simulink model "Exercise1"  (R2025b)
settings: Solver=FixedStepAuto  StartTime=0.0  StopTime=300  FixedStep=Ts  RelTol=1e-3
values from neighbouring files (symbols this model uses):
  a = 0.923    [VehicleParameters.m]
  b = 1.376    [VehicleParameters.m]
  CMy = 0.1    [VehicleParameters.m]
  Cx = Cx0    [Exercise_Workbook.m]    (also in VehicleParameters.m = 0.33)
  Cz = 0.2    [VehicleParameters.m]
  eta_t = 0.93    [VehicleParameters.m]
  f0 = 0.011    [VehicleParameters.m]
  g = 9.81    [VehicleParameters.m]
  gear_vec = i_g    [Exercise_Workbook.m]
  ha = 0    [Exercise_Workbook.m]
  hb = 0.5    [Exercise_Workbook.m]
  hc = 0    [Exercise_Workbook.m]
  hG = 0.6    [VehicleParameters.m]
  i_f = 3.438    [VehicleParameters.m]
  i_g = [3.909 , 2.157 , 1.48 , 1.121 , 0.897]    [VehicleParameters.m]
  Je = 0.088    [VehicleParameters.m]
  Jt = 0.05    [VehicleParameters.m]
  Jw = 0.59    [VehicleParameters.m]
  K = 2.6e-8    (= 2.6e-08)    [VehicleParameters.m]
  l = a+b    (= 2.299)    [VehicleParameters.m]
  m = m0    [Exercise_Workbook.m]    (also in VehicleParameters.m = 1020)
  mu_vec = mu_wet    [Exercise_Workbook.m]
  n_shiftdown = 140    [Exercise_Workbook.m]
  n_shiftup = 450    [Exercise_Workbook.m]
  n_vec = n_compact    [Exercise_Workbook.m]
  omega0 = V0/Re    [Exercise_Workbook.m]
  Rc = Re    (= 0.279)    [VehicleParameters.m]
  ro = 1.2    [VehicleParameters.m]
  S = 2.04    [VehicleParameters.m]
  sigma_vec = sigma    [Exercise_Workbook.m]
  startingGear = 5    [Exercise_Workbook.m]
  t_pedalAct = 0.2    [Exercise_Workbook.m]
  t_shifting = 0.6    [Exercise_Workbook.m]
  T_vec = T_compact    [Exercise_Workbook.m]
  tau_f = 1./i_f    (= 0.290866783013)    [VehicleParameters.m]
  Tbf_max = TbTot/(1 + 1/Kb)    (= 2099.0990991)    [Exercise_Workbook.m]
  Tbr_max = Tbf_max/Kb    (= 900.900900901)    [Exercise_Workbook.m]
  Tc_max = 1.2*Te_max    (= 126)    [VehicleParameters.m]
  Traction = 2    [Exercise_Workbook.m]    (also in VehicleParameters.m = 1)
  Ts = 1e-3    (= 0.001)    [Exercise_Workbook.m]
  V0 = 80/3.6    (= 22.2222222222)    [Exercise_Workbook.m]
libraries: simulink x2
settings Model: Creator=Alberto  LastModifiedBy=denni
settings OptimizationCC: ReuseModelBlockBuffer=off
settings RTWCC: GPUComputeCapability=3.5

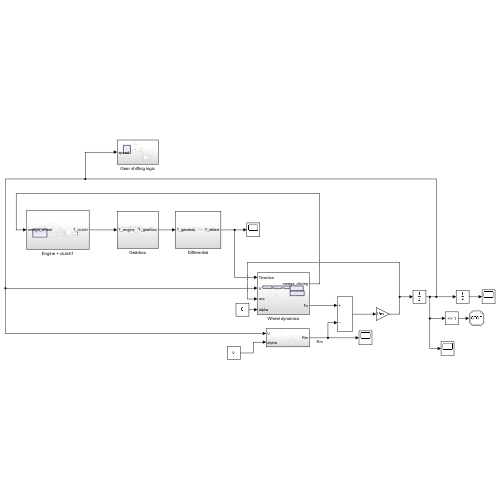
[thumbnail: Simulink's stored preview of the top-level diagram]
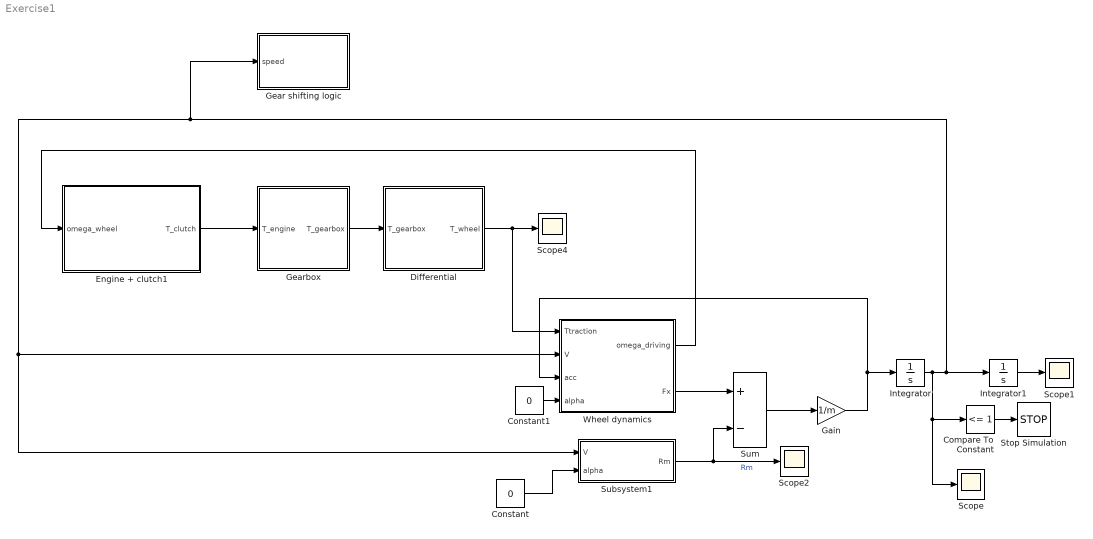
== system Exercise1 ==
  Compare To Constant : simulink/Logic and Bit Operations/Compare To Constant  relop=<=  const=1  OutDataTypeStr=boolean
  Constant : Constant  Value=0
  Constant1 : Constant  Value=0
  Differential : Subsystem
  Engine + clutch1 : Subsystem
  Gain : Gain  Gain=1/m
  Gear shifting logic : Subsystem
  Gearbox : Subsystem
  Integrator : Integrator  InitialCondition=V0
  Integrator1 : Integrator
  Scope{,1..2,4} (4 alike) : Scope
      Scope settings: ActiveDisplayYMinimum=-3.29722  ActiveDisplayYMaximum=4.84775  DataLoggingVariableName=Speed
      Scope1 settings: ActiveDisplayYMinimum=-21.94682  ActiveDisplayYMaximum=197.52142  DataLoggingVariableName=Distance
      Scope2 settings: ActiveDisplayYMinimum=-3.670379518302145E+57  ActiveDisplayYMaximum=3.3033415664719314E+58  DataLoggingVariableName=ScopeData3
      Scope4 settings: ActiveDisplayYMinimum=-433.41267  ActiveDisplayYMaximum=536.48619  DataLoggingVariableName=ScopeData9
  Stop Simulation : Stop
  Subsystem1 : Subsystem
  Sum : Sum  Inputs=+-
  Wheel dynamics : Subsystem
  wires:
  Integrator/1 -> Compare To Constant/1, Scope/1, Gear shifting logic/1(speed), Wheel dynamics/2(V), Subsystem1/1(V), Integrator1/1
  Wheel dynamics/2(Fx) -> Sum/1
  Subsystem1/1(Rm) -> Scope2/1, Sum/2  "Rm"
  Constant/1 -> Subsystem1/2(alpha)
  Sum/1 -> Gain/1
  Gain/1 -> Wheel dynamics/3(acc), Integrator/1
  Integrator1/1 -> Scope1/1
  Compare To Constant/1 -> Stop Simulation/1
  Constant1/1 -> Wheel dynamics/4(alpha)
  Gearbox/1(T_gearbox) -> Differential/1(T_gearbox)
  Differential/1(T_wheel) -> Wheel dynamics/1(Ttraction), Scope4/1
  Engine + clutch1/1(T_clutch) -> Gearbox/1(T_engine)
  Wheel dynamics/1(omega_driving) -> Engine + clutch1/1(omega_wheel)

== system Exercise1/Differential ==
  T_gearbox : Inport
  Gain3 : Gain  Gain=0.5*i_f
  T_wheel : Outport
  wires:
  T_gearbox/1 -> Gain3/1
  Gain3/1 -> T_wheel/1

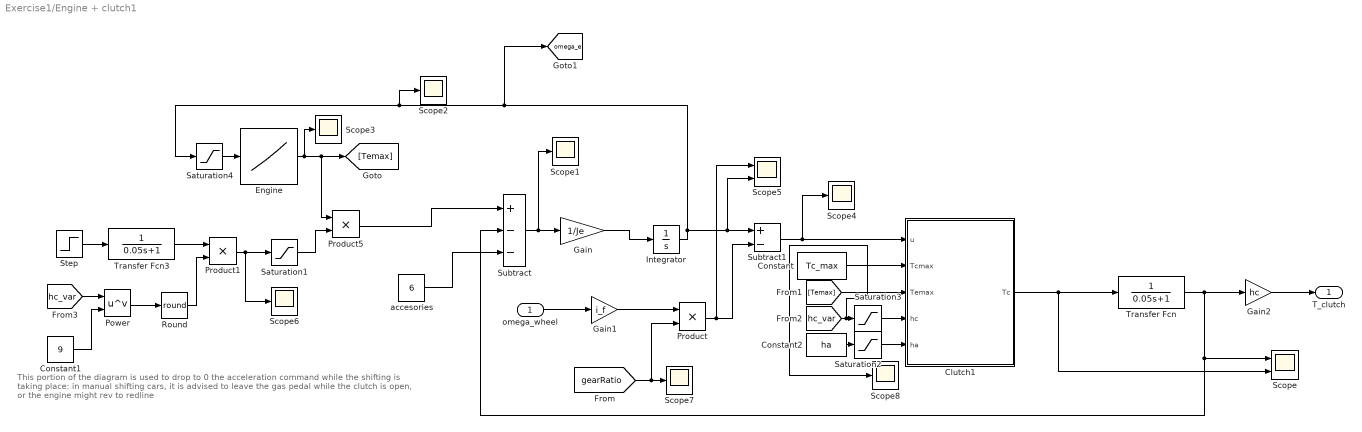
== system Exercise1/Engine + clutch1 ==
  note: This portion of the diagram is used to drop to 0 the acceleration command while the shifting is taking place: in manual shifting cars, it is advised to leave the gas pedal while the clutch is open, or the engine might rev to redline
  omega_wheel : Inport
  Clutch1 : MATLAB Function  TreatAsAtomicUnit=on
  Constant : Constant  Value=Tc_max
  Constant1 : Constant  Value=9
  Constant2 : Constant  Value=ha
  Engine : Lookup_n-D  NumberOfTableDimensions=1  BreakpointsForDimension1=n_vec  Table=T_vec  InternalRulePriority=Speed  RndMeth=Simplest
  Gain : Gain  Gain=1/Je
  Gain1 : Gain  Gain=i_f
  Gain2 : Gain  Gain=hc
  Integrator : Integrator  InitialCondition=omega0*i_g(5)*i_f
  Power : Math  Operator=pow
  Product : Product
  Product1 : Product
  Product5 : Product
  Round : Rounding  Operator=round
  Saturation1 : Saturate  UpperLimit=1  LowerLimit=0
  Saturation2 : Saturate  UpperLimit=1  LowerLimit=0
  Saturation3 : Saturate  UpperLimit=1  LowerLimit=0
  Saturation4 : Saturate  UpperLimit=max(n_vec)  LowerLimit=min(n_vec)
  Scope : Scope  NumInputPorts=2
      settings: ActiveDisplayYMinimum=-157.5  ActiveDisplayYMaximum=157.5  DataLoggingVariableName=ScopeData11
  Scope{1..4,6..8} (7 alike) : Scope
      Scope1 settings: ActiveDisplayYMinimum=-1.4800422611786087E+307  ActiveDisplayYMaximum=1.6444914013095649E+306  DataLoggingVariableName=ScopeData5
      Scope2 settings: ActiveDisplayYMinimum=-234.98976  ActiveDisplayYMaximum=2163.66995  DataLoggingVariableName=ScopeData6
      Scope3 settings: ActiveDisplayYMinimum=42.3058  ActiveDisplayYMaximum=110.8549  DataLoggingVariableName=ScopeData7
      Scope4 settings: ActiveDisplayYMinimum=-233.77506  ActiveDisplayYMaximum=296.88623  DataLoggingVariableName=ScopeData9
      Scope6 settings: ActiveDisplayYMinimum=-1  ActiveDisplayYMaximum=1
      Scope7 settings: ActiveDisplayYMinimum=3.85912  ActiveDisplayYMaximum=3.95022  DataLoggingVariableName=ScopeData2
      Scope8 settings: ActiveDisplayYMinimum=-0.11944  ActiveDisplayYMaximum=1.12438  DataLoggingVariableName=ScopeData2
  Scope5 : Scope  NumInputPorts=2
      settings: ActiveDisplayYMinimum=-55.03177  ActiveDisplayYMaximum=558.78238  DataLoggingVariableName=ScopeData10
  Step : Step  Time=0  After=ha  SampleTime=0
  Subtract : Sum  Inputs=+--
  Subtract1 : Sum  Inputs=+-
  Transfer Fcn : TransferFcn  Denominator=[0.05 1]
  Transfer Fcn3 : TransferFcn  Denominator=[0.05 1]
  accesories : Constant  Value=6
  T_clutch : Outport
  tag scope: omega_e=global
  wires:
  Engine/1 -> Scope3/1, [Temax], Product5/1
  Product5/1 -> Subtract/1
  Saturation1/1 -> Product5/2
  Subtract/1 -> Scope1/1, Gain/1
  Gain/1 -> Integrator/1
  omega_wheel/1 -> Gain1/1
  Gain1/1 -> Product/1
  [gearRatio] -> Product/2, Scope7/1
  Product/1 -> Scope5/1, Subtract1/2
  Subtract1/1 -> Clutch1/1(u), Scope4/1
  Constant/1 -> Clutch1/2(Tcmax)
  [Temax] -> Clutch1/3(Temax)
  Saturation3/1 -> Clutch1/4(hc)
  [hc_var] -> Scope8/1, Saturation3/1
  Constant2/1 -> Saturation2/1
  Saturation2/1 -> Clutch1/5(ha)
  Integrator/1 -> [omega_e], Saturation4/1, Scope2/1, Scope5/2, Subtract1/1
  Transfer Fcn3/1 -> Product1/1
  Product1/1 -> Scope6/1, Saturation1/1
  Round/1 -> Product1/2
  [hc_var] -> Power/1
  Power/1 -> Round/1
  Constant1/1 -> Power/2
  Clutch1/1(Tc) -> Scope/2, Transfer Fcn/1
  Step/1 -> Transfer Fcn3/1
  Saturation4/1 -> Engine/1
  accesories/1 -> Subtract/3
  Gain2/1 -> T_clutch/1
  Transfer Fcn/1 -> Subtract/2, Scope/1, Gain2/1

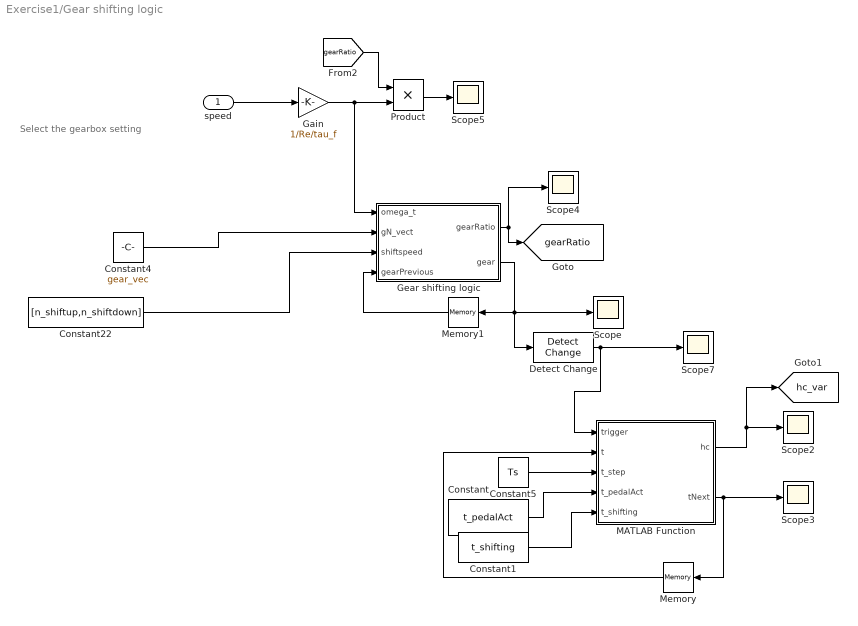
== system Exercise1/Gear shifting logic ==
  note: Select the gearbox setting
  speed : Inport
  Constant : Constant  Value=t_pedalAct
  Constant1 : Constant  Value=t_shifting
  Constant22 : Constant  Value=[n_shiftup,n_shiftdown]
  Constant4 : Constant  Value=gear_vec  SampleTime=Ts
  Constant5 : Constant  Value=Ts
  Detect Change : simulink/Logic and Bit Operations/Detect Change  vinit=0  OutDataTypeStr=boolean
  Gain : Gain  Gain=1/Re/tau_f
  Gear shifting logic : MATLAB Function  TreatAsAtomicUnit=on
  MATLAB Function : MATLAB Function  TreatAsAtomicUnit=on
  Memory : Memory
  Memory1 : Memory  InitialCondition=startingGear
  Product : Product
  Scope{,2..5,7} (6 alike) : Scope
      Scope settings: ActiveDisplayYMinimum=0.5  ActiveDisplayYMaximum=5.5
      Scope2 settings: ActiveDisplayYMinimum=-0.11944  ActiveDisplayYMaximum=1.12438  DataLoggingVariableName=ScopeData2
      Scope3 settings: ActiveDisplayYMinimum=-0.6325  ActiveDisplayYMaximum=5.6925  DataLoggingVariableName=ScopeData3
      Scope4 settings: ActiveDisplayYMinimum=0.7725  ActiveDisplayYMaximum=4.2575  DataLoggingVariableName=ScopeData8
      Scope5 settings: ActiveDisplayYMinimum=-25.93069  ActiveDisplayYMaximum=467.45559
      Scope7 settings: ActiveDisplayYMinimum=-0.125  ActiveDisplayYMaximum=1.125  DataLoggingVariableName=ScopeData2
  tag scope: gearRatio=global, hc_var=global
  wires:
  Gear shifting logic/1(gearRatio) -> [gearRatio], Scope4/1
  Constant22/1 -> Gear shifting logic/3(shiftspeed)
  Gear shifting logic/2(gear) -> Scope/1, Memory1/1, Detect Change/1
  Detect Change/1 -> MATLAB Function/1(trigger), Scope7/1
  MATLAB Function/2(tNext) -> Scope3/1, Memory/1
  Memory/1 -> MATLAB Function/2(t)
  MATLAB Function/1(hc) -> [hc_var], Scope2/1
  Memory1/1 -> Gear shifting logic/4(gearPrevious)
  Constant/1 -> MATLAB Function/4(t_pedalAct)
  Constant1/1 -> MATLAB Function/5(t_shifting)
  Constant5/1 -> MATLAB Function/3(t_step)
  speed/1 -> Gain/1
  Gain/1 -> Product/2, Gear shifting logic/1(omega_t)
  Constant4/1 -> Gear shifting logic/2(gN_vect)
  [gearRatio] -> Product/1
  Product/1 -> Scope5/1

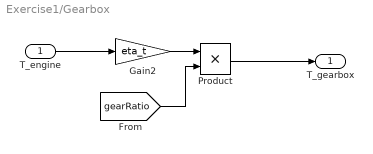
== system Exercise1/Gearbox ==
  T_engine : Inport
  Gain2 : Gain  Gain=eta_t
  Product : Product
  T_gearbox : Outport
  wires:
  Gain2/1 -> Product/1
  T_engine/1 -> Gain2/1
  Product/1 -> T_gearbox/1
  [gearRatio] -> Product/2

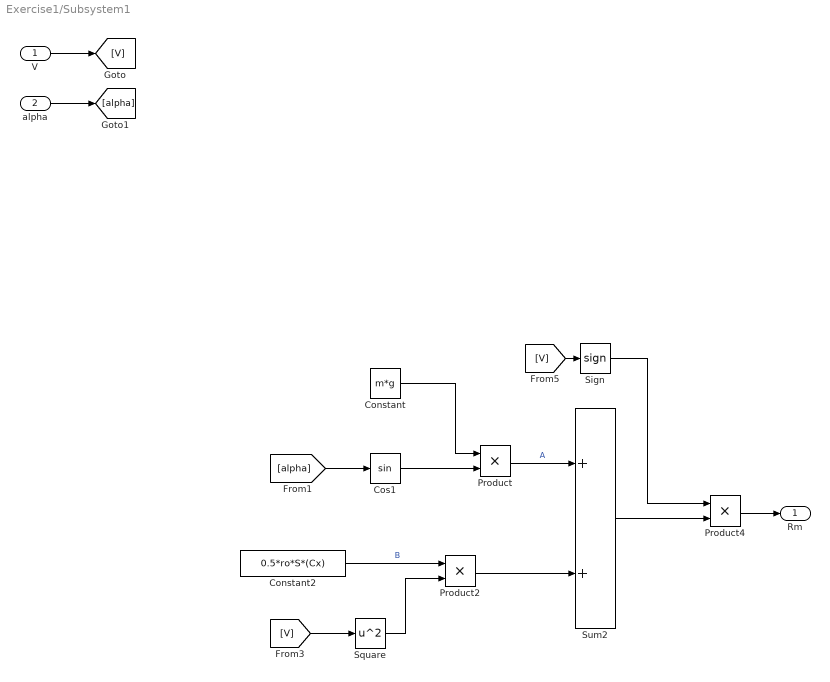
== system Exercise1/Subsystem1 ==
  V : Inport
  alpha : Inport  Port=2
  Constant : Constant  Value=m*g
  Constant2 : Constant  Value=0.5*ro*S*(Cx)
  Cos1 : Trigonometry
  Product : Product
  Product2 : Product
  Product4 : Product
  Sign : Signum
  Square : Math  Operator=square
  Sum2 : Sum
  Rm : Outport
  wires:
  V/1 -> [V]
  alpha/1 -> [alpha]
  [alpha] -> Cos1/1
  Cos1/1 -> Product/2
  Constant/1 -> Product/1
  Product/1 -> Sum2/1  "A"
  Constant2/1 -> Product2/1  "B"
  [V] -> Square/1
  Square/1 -> Product2/2
  Product2/1 -> Sum2/2
  Product4/1 -> Rm/1
  Sum2/1 -> Product4/2
  [V] -> Sign/1
  Sign/1 -> Product4/1

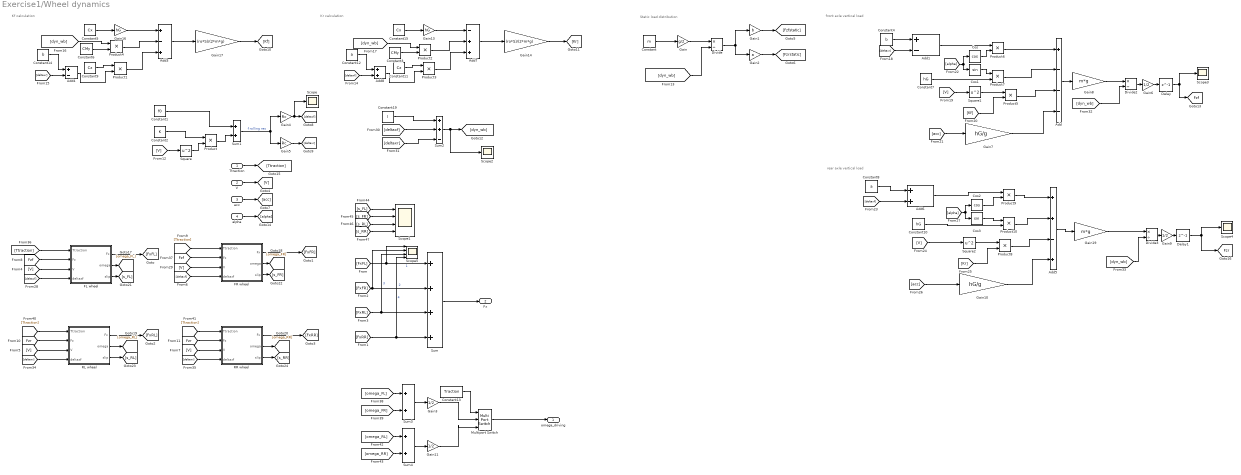
== system Exercise1/Wheel dynamics ==
  note: Static load distribution
  note: Kr calculation
  note: Kf calculation
  note: front axle vertical load
  note: rear axle vertical load
  Ttraction : Inport
  V : Inport  Port=2
  acc : Inport  Port=3
  alpha : Inport  Port=4
  Add : Sum  Inputs=+---
  Add1 : Sum  Inputs=+-
  Add3 : Sum  Inputs=+-+
  Add4 : Sum  Inputs=+-
  Add5 : Sum  Inputs=++-+
  Add6 : Sum
  Add7 : Sum  Inputs=-++
  Add8 : Sum
  Constant : Constant  Value=m
  Constant1 : Constant  Value=f0
  Constant10 : Constant  Value=hG
  Constant11 : Constant  Value=Cz
  Constant12 : Constant  Value=a
  Constant13 : Constant  Value=Traction
  Constant14 : Constant  Value=b
  Constant15 : Constant  Value=Cx
  Constant19 : Constant  Value=l
  Constant2 : Constant  Value=K
  Constant3 : Constant  Value=CMy
  Constant4 : Constant  Value=b
  Constant5 : Constant  Value=Cx
  Constant6 : Constant  Value=CMy
  Constant7 : Constant  Value=hG
  Constant8 : Constant  Value=a
  Constant9 : Constant  Value=Cz
  Cos : Trigonometry  Operator=cos
  Cos1 : Trigonometry
  Cos2 : Trigonometry  Operator=cos
  Cos3 : Trigonometry
  Delay : Delay  DelayLength=1  InitialCondition=m*g*b/l/2
  Delay1 : Delay  DelayLength=1  InitialCondition=m*g*a/l/2
  Divide : Product  Inputs=*/
  Divide2 : Product  Inputs=*/
  Divide3 : Product  Inputs=*/
  FL wheel : Subsystem
  FR wheel : Subsystem
  Gain : Gain  Gain=g/2
  Gain1 : Gain  Gain=b
  Gain10 : Gain  Gain=hG/g
  Gain{3,6,9,11} (4 alike) : Gain  Gain=1/2
  Gain13 : Gain  Gain=hG
  Gain14 : Gain  Gain=(ro*S)/(2*m*g)
  Gain16 : Gain  Gain=hG
  Gain17 : Gain  Gain=(ro*S)/(2*m*g)
  Gain19 : Gain  Gain=m*g
  Gain2 : Gain  Gain=a
  Gain4 : Gain  Gain=Rc
  Gain5 : Gain  Gain=Rc
  Gain7 : Gain  Gain=hG/g
  Gain8 : Gain  Gain=m*g
  Multiport Switch : MultiPortSwitch  Inputs=2  SaturateOnIntegerOverflow=off  InputSameDT=off
  Product{,1..10} (11 alike) : Product
  RL wheel : Subsystem
  RR wheel : Subsystem
  Scope{,2..4} (4 alike) : Scope
      Scope settings: ActiveDisplayYMinimum=0.003067  ActiveDisplayYMaximum=0.003086  DataLoggingVariableName=ScopeData2
      Scope2 settings: ActiveDisplayYMinimum=1.299  ActiveDisplayYMaximum=3.299  DataLoggingVariableName=ScopeData4
      Scope3 settings: ActiveDisplayYMinimum=2850.0417  ActiveDisplayYMaximum=3925.07758
      Scope4 settings: ActiveDisplayYMinimum=1017.63681  ActiveDisplayYMaximum=2054.66126  DataLoggingVariableName=ScopeData2
  Scope1 : Scope  NumInputPorts=4
      settings: ActiveDisplayYMinimum=-0.57113  ActiveDisplayYMaximum=0.11334  DataLoggingVariableName=slip
  Scope5 : Scope  NumInputPorts=4
      settings: ActiveDisplayYMinimum=-3828.18796  ActiveDisplayYMaximum=425.35422  DataLoggingVariableName=ScopeData3
  Square : Math  Operator=square
  Square1 : Math  Operator=square
  Square2 : Math  Operator=square
  Sum : Sum  Inputs=++++
  Sum1 : Sum
  Sum2 : Sum  Inputs=++-
  Sum3 : Sum
  Sum4 : Sum
  omega_driving : Outport
  Fx : Outport  Port=2
  tag scope: Fzf=global, Fzr=global
  wires:
  FL wheel/1(Fx) -> [FxFL]
  [V] -> RR wheel/3(V)
  [FxRL] -> Scope5/3, Sum/3  "3"
  V/1 -> [V]
  Sum/1 -> Fx/1
  RR wheel/1(Fx) -> [FxRR]
  [FxRR] -> Scope5/4, Sum/4  "4"
  [FxFL] -> Scope5/1, Sum/1  "1"
  FR wheel/1(Fx) -> [FxFR]
  [V] -> FL wheel/3(V)
  [V] -> RL wheel/3(V)
  RL wheel/1(Fx) -> [FxRL]
  [Fzf] -> FL wheel/2(Fz)
  Constant/1 -> Gain/1
  Gain1/1 -> [Fzfstatic]
  Gain2/1 -> [Fzrstatic]
  [Fzr] -> RL wheel/2(Fz)
  [Fzr] -> RR wheel/2(Fz)
  acc/1 -> [acc]
  [V] -> Square/1
  Constant2/1 -> Product/1
  Square/1 -> Product/2
  Constant1/1 -> Sum1/1
  Product/1 -> Sum1/2
  Sum1/1 -> Gain5/1, Gain4/1  "f rolling res"
  Gain4/1 -> Scope/1, [deltaxf]
  Gain5/1 -> [deltaxr]
  Constant19/1 -> Sum2/1
  [deltaxr] -> Sum2/3
  Sum2/1 -> Scope2/1, [dyn_wb]
  [deltaxf] -> Sum2/2
  Gain/1 -> Divide/1
  [dyn_wb] -> Divide/2
  Divide/1 -> Gain2/1, Gain1/1
  Add4/1 -> Product1/2
  Gain17/1 -> [Kf]
  Product1/1 -> Add3/3
  Product3/1 -> Add7/3
  Constant5/1 -> Gain16/1
  Add8/1 -> Product3/2
  Constant12/1 -> Add8/1
  Constant15/1 -> Gain13/1
  Product2/1 -> Add7/2
  Product4/1 -> Add3/2
  Add3/1 -> Gain17/1
  Constant9/1 -> Product1/1
  Constant11/1 -> Product3/1
  [deltaxr] -> Add4/2
  Add7/1 -> Gain14/1
  Gain14/1 -> [Kr]
  [deltaxf] -> Add8/2
  Gain13/1 -> Add7/1
  Gain16/1 -> Add3/1
  Constant14/1 -> Add4/1
  Constant6/1 -> Product4/2
  [dyn_wb] -> Product4/1
  Constant3/1 -> Product2/2
  [dyn_wb] -> Product2/1
  Product5/1 -> Add/3
  Gain7/1 -> Add/4
  Square1/1 -> Product5/1
  Constant4/1 -> Add1/1
  [Kf] -> Product5/2
  Product7/1 -> Add/2
  Add1/1 -> Product6/1
  Constant7/1 -> Product7/2
  [dyn_wb] -> Divide2/2
  [V] -> Square1/1
  [acc] -> Gain7/1
  Gain8/1 -> Divide2/1
  Product6/1 -> Add/1
  Add/1 -> Gain8/1
  [deltaxr] -> Add1/2
  Cos/1 -> Product6/2
  Cos1/1 -> Product7/1
  alpha/1 -> [alpha]
  [alpha] -> Cos/1, Cos1/1
  Divide2/1 -> Gain6/1
  [V] -> Square2/1
  [acc] -> Gain10/1
  Constant10/1 -> Product10/2
  Add5/1 -> Gain19/1
  Constant8/1 -> Add6/1
  Product9/1 -> Add5/1
  [dyn_wb] -> Divide3/2
  Add6/1 -> Product9/1
  Square2/1 -> Product8/1
  Product8/1 -> Add5/3
  [Kr] -> Product8/2
  Gain19/1 -> Divide3/1
  Gain10/1 -> Add5/4
  Product10/1 -> Add5/2
  [deltaxf] -> Add6/2
  [alpha] -> Cos2/1, Cos3/1
  Cos2/1 -> Product9/2
  Cos3/1 -> Product10/1
  Divide3/1 -> Gain9/1
  Gain6/1 -> Delay/1
  Delay/1 -> [Fzf], Scope3/1
  Gain9/1 -> Delay1/1
  [deltaxf] -> FL wheel/4(deltaxf)
  [deltaxr] -> RL wheel/4(deltaxf)
  [deltaxr] -> RR wheel/4(deltaxf)
  Delay1/1 -> [Fzr], Scope4/1
  Ttraction/1 -> [Ttraction]
  [Ttraction] -> FL wheel/1(Ttraction)
  [Ttraction] -> FR wheel/1(Ttraction)
  [V] -> FR wheel/3(V)
  [deltaxf] -> FR wheel/4(deltaxf)
  [Fzf] -> FR wheel/2(Fz)
  FL wheel/2(omega) -> [omega_FL]
  FR wheel/2(omega) -> [omega_FR]
  [omega_FL] -> Sum3/1
  [omega_FR] -> Sum3/2
  Sum3/1 -> Gain3/1
  [Ttraction] -> RL wheel/1(Ttraction)
  RL wheel/2(omega) -> [omega_RL]
  [Ttraction] -> RR wheel/1(Ttraction)
  RR wheel/2(omega) -> [omega_RR]
  Sum4/1 -> Gain11/1
  [omega_RR] -> Sum4/2
  [omega_RL] -> Sum4/1
  Gain3/1 -> Multiport Switch/2
  Gain11/1 -> Multiport Switch/3
  Constant13/1 -> Multiport Switch/1
  Multiport Switch/1 -> omega_driving/1
  FL wheel/3(slip) -> [s_FL]
  FR wheel/3(slip) -> [s_FR]
  RL wheel/3(slip) -> [s_RL]
  RR wheel/3(slip) -> [s_RR]
  [s_FL] -> Scope1/1
  [s_FR] -> Scope1/2
  [s_RL] -> Scope1/3
  [s_RR] -> Scope1/4
  [FxFR] -> Scope5/2, Sum/2  "2"

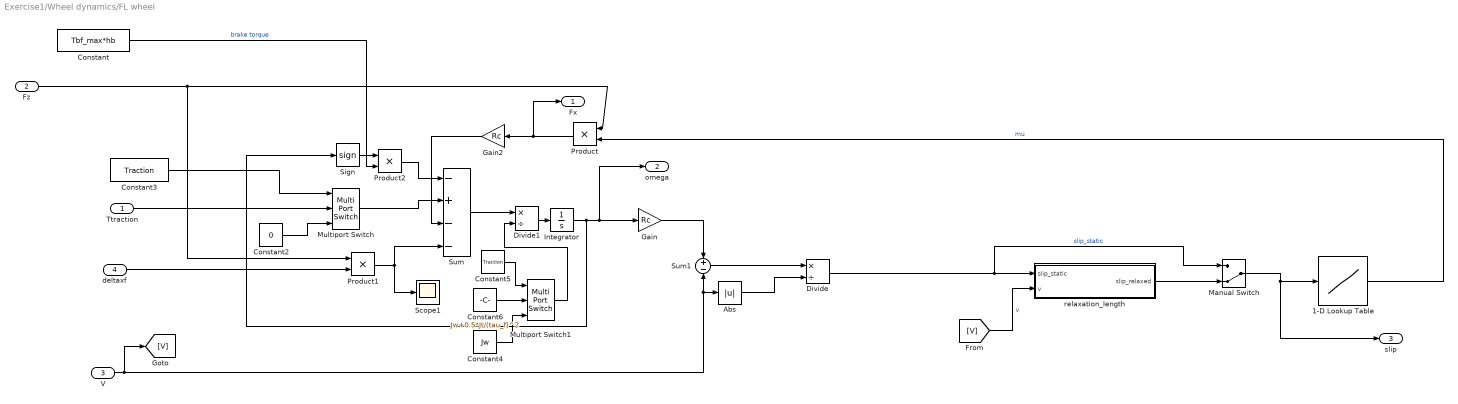
== system Exercise1/Wheel dynamics/FL wheel ==
  Ttraction : Inport
  Fz : Inport  Port=2
  V : Inport  Port=3
  deltaxf : Inport  Port=4
  1-D Lookup Table : Lookup_n-D  NumberOfTableDimensions=1  BreakpointsForDimension1=sigma_vec  Table=mu_vec  InternalRulePriority=Speed  RndMeth=Simplest
  Abs : Abs  SaturateOnIntegerOverflow=off
  Constant : Constant  Value=Tbf_max*hb
  Constant2 : Constant  Value=0
  Constant3 : Constant  Value=Traction
  Constant4 : Constant  Value=Jw
  Constant5 : Constant  Value=Traction
  Constant6 : Constant  Value=Jw+0.5*Jt/(tau_f)^2
  Divide : Product  Inputs=*/
  Divide1 : Product  Inputs=*/
  Gain : Gain  Gain=Rc
  Gain2 : Gain  Gain=Rc
  Integrator : Integrator  InitialCondition=omega0  LimitOutput=on  LowerSaturationLimit=0
  Manual Switch : ManualSwitch  CurrentSetting=0
  Multiport Switch : MultiPortSwitch  Inputs=2  SaturateOnIntegerOverflow=off  InputSameDT=off
  Multiport Switch1 : MultiPortSwitch  Inputs=2  SaturateOnIntegerOverflow=off  InputSameDT=off
  Product : Product
  Product1 : Product
  Product2 : Product
  Scope1 : Scope
      settings: ActiveDisplayYMinimum=4.6511  ActiveDisplayYMaximum=15.35009  DataLoggingVariableName=ScopeData8
  Sign : Signum
  Sum : Sum  Inputs=-+--
  Sum1 : Sum  Inputs=+-
  relaxation_length : Subsystem
  Fx : Outport
  omega : Outport  Port=2
  slip : Outport  Port=3
  wires:
  Gain/1 -> Sum1/1
  Gain2/1 -> Sum/3
  V/1 -> [V], Abs/1, Sum1/2
  Product/1 -> Fx/1, Gain2/1
  1-D Lookup Table/1 -> Product/2  "mu"
  Integrator/1 -> Sign/1, omega/1, Gain/1
  Sum1/1 -> Divide/1
  Divide/1 -> relaxation_length/1(slip_static), Manual Switch/1  "slip_static"
  Fz/1 -> Product/1, Product1/1
  Abs/1 -> Divide/2
  deltaxf/1 -> Product1/2
  Product1/1 -> Sum/4, Scope1/1
  Multiport Switch/1 -> Sum/2
  Constant2/1 -> Multiport Switch/3
  Ttraction/1 -> Multiport Switch/2
  Constant3/1 -> Multiport Switch/1
  Constant5/1 -> Multiport Switch1/1
  Multiport Switch1/1 -> Divide1/2
  Sum/1 -> Divide1/1
  Constant4/1 -> Multiport Switch1/3
  Constant6/1 -> Multiport Switch1/2
  Divide1/1 -> Integrator/1
  Sign/1 -> Product2/1
  Constant/1 -> Product2/2  "brake torque"
  Product2/1 -> Sum/1
  [V] -> relaxation_length/2(v)  "v"
  Manual Switch/1 -> slip/1, 1-D Lookup Table/1
  relaxation_length/1(slip_relaxed) -> Manual Switch/2

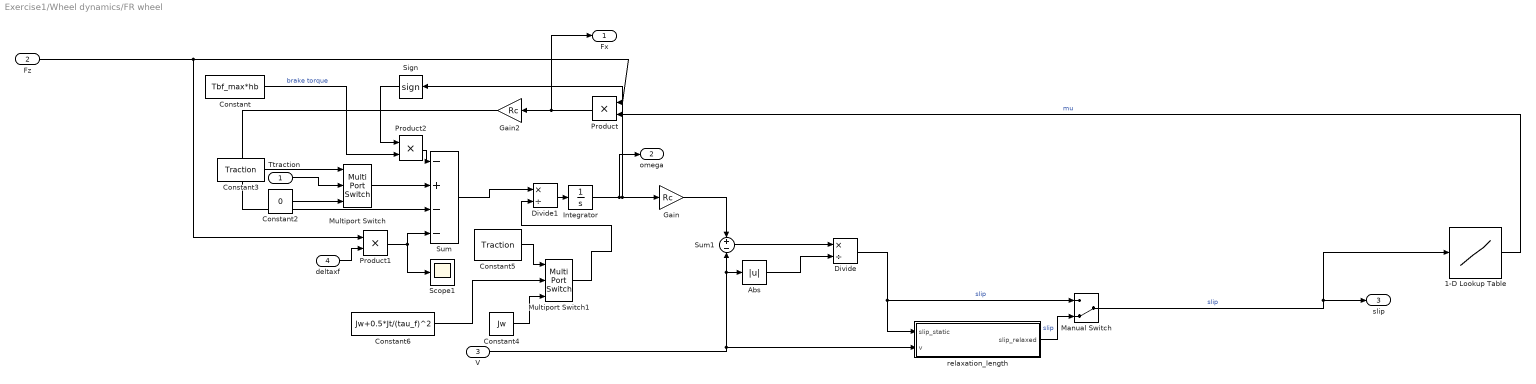
== system Exercise1/Wheel dynamics/FR wheel ==
  Ttraction : Inport
  Fz : Inport  Port=2
  V : Inport  Port=3
  deltaxf : Inport  Port=4
  1-D Lookup Table : Lookup_n-D  NumberOfTableDimensions=1  BreakpointsForDimension1=sigma_vec  Table=mu_vec  InternalRulePriority=Speed  RndMeth=Simplest
  Abs : Abs  SaturateOnIntegerOverflow=off
  Constant : Constant  Value=Tbf_max*hb
  Constant2 : Constant  Value=0
  Constant3 : Constant  Value=Traction
  Constant4 : Constant  Value=Jw
  Constant5 : Constant  Value=Traction
  Constant6 : Constant  Value=Jw+0.5*Jt/(tau_f)^2
  Divide : Product  Inputs=*/
  Divide1 : Product  Inputs=*/
  Gain : Gain  Gain=Rc
  Gain2 : Gain  Gain=Rc
  Integrator : Integrator  InitialCondition=omega0  LimitOutput=on  LowerSaturationLimit=0
  Manual Switch : ManualSwitch  CurrentSetting=0
  Multiport Switch : MultiPortSwitch  Inputs=2  SaturateOnIntegerOverflow=off  InputSameDT=off
  Multiport Switch1 : MultiPortSwitch  Inputs=2  SaturateOnIntegerOverflow=off  InputSameDT=off
  Product : Product
  Product1 : Product
  Product2 : Product
  Scope1 : Scope
      settings: ActiveDisplayYMinimum=4.6511  ActiveDisplayYMaximum=15.35009  DataLoggingVariableName=ScopeData8
  Sign : Signum
  Sum : Sum  Inputs=-+--
  Sum1 : Sum  Inputs=+-
  relaxation_length : Subsystem
  Fx : Outport
  omega : Outport  Port=2
  slip : Outport  Port=3
  wires:
  Product2/1 -> Sum/1
  Constant/1 -> Product2/2  "brake torque"
  Sign/1 -> Product2/1
  Divide1/1 -> Integrator/1
  Constant6/1 -> Multiport Switch1/2
  Constant4/1 -> Multiport Switch1/3
  Sum/1 -> Divide1/1
  Multiport Switch1/1 -> Divide1/2
  Constant5/1 -> Multiport Switch1/1
  Constant3/1 -> Multiport Switch/1
  Ttraction/1 -> Multiport Switch/2
  Constant2/1 -> Multiport Switch/3
  Multiport Switch/1 -> Sum/2
  Product1/1 -> Scope1/1, Sum/4
  deltaxf/1 -> Product1/2
  Abs/1 -> Divide/2
  Fz/1 -> Product1/1, Product/1
  Manual Switch/1 -> 1-D Lookup Table/1, slip/1  "slip"
  Sum1/1 -> Divide/1
  Integrator/1 -> Sign/1, Gain/1, omega/1
  1-D Lookup Table/1 -> Product/2  "mu"
  Product/1 -> Gain2/1, Fx/1
  V/1 -> relaxation_length/2(v), Sum1/2, Abs/1
  Gain2/1 -> Sum/3
  Gain/1 -> Sum1/1
  Divide/1 -> relaxation_length/1(slip_static), Manual Switch/1  "slip"
  relaxation_length/1(slip_relaxed) -> Manual Switch/2  "slip"

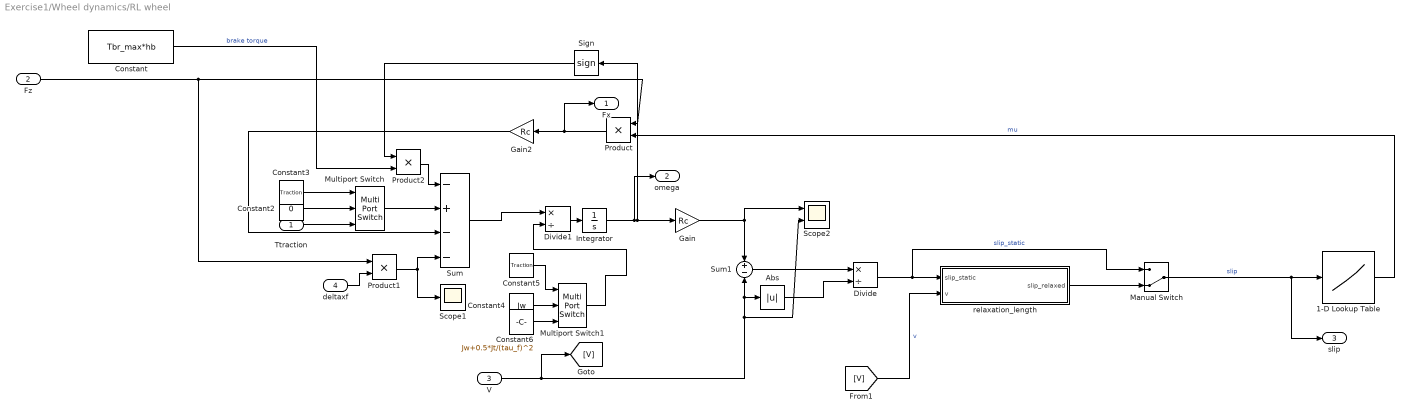
== system Exercise1/Wheel dynamics/RL wheel ==
  Ttraction : Inport
  Fz : Inport  Port=2
  V : Inport  Port=3
  deltaxf : Inport  Port=4
  1-D Lookup Table : Lookup_n-D  NumberOfTableDimensions=1  BreakpointsForDimension1=sigma_vec  Table=mu_vec  InternalRulePriority=Speed  RndMeth=Simplest
  Abs : Abs  SaturateOnIntegerOverflow=off
  Constant : Constant  Value=Tbr_max*hb
  Constant2 : Constant  Value=0
  Constant3 : Constant  Value=Traction
  Constant4 : Constant  Value=Jw
  Constant5 : Constant  Value=Traction
  Constant6 : Constant  Value=Jw+0.5*Jt/(tau_f)^2
  Divide : Product  Inputs=*/
  Divide1 : Product  Inputs=*/
  Gain : Gain  Gain=Rc
  Gain2 : Gain  Gain=Rc
  Integrator : Integrator  InitialCondition=omega0  LimitOutput=on  LowerSaturationLimit=0
  Manual Switch : ManualSwitch  CurrentSetting=0
  Multiport Switch : MultiPortSwitch  Inputs=2  SaturateOnIntegerOverflow=off  InputSameDT=off
  Multiport Switch1 : MultiPortSwitch  Inputs=2  SaturateOnIntegerOverflow=off  InputSameDT=off
  Product : Product
  Product1 : Product
  Product2 : Product
  Scope1 : Scope
      settings: ActiveDisplayYMinimum=1.38626  ActiveDisplayYMaximum=12.08532  DataLoggingVariableName=ScopeData8
  Scope2 : Scope  NumInputPorts=2
      settings: ActiveDisplayYMinimum=-5.63176  ActiveDisplayYMaximum=50.62575  DataLoggingVariableName=ScopeData6
  Sign : Signum
  Sum : Sum  Inputs=-+--
  Sum1 : Sum  Inputs=+-
  relaxation_length : Subsystem
  Fx : Outport
  omega : Outport  Port=2
  slip : Outport  Port=3
  wires:
  Gain/1 -> Sum1/1, Scope2/1
  Gain2/1 -> Sum/3
  V/1 -> [V], Sum1/2, Abs/1, Scope2/2
  Product/1 -> Fx/1, Gain2/1
  1-D Lookup Table/1 -> Product/2  "mu"
  Integrator/1 -> Sign/1, Gain/1, omega/1
  Sum1/1 -> Divide/1
  Manual Switch/1 -> slip/1, 1-D Lookup Table/1  "slip"
  Fz/1 -> Product/1, Product1/1
  deltaxf/1 -> Product1/2
  Product1/1 -> Sum/4, Scope1/1
  Multiport Switch/1 -> Sum/2
  Constant3/1 -> Multiport Switch/1
  Constant5/1 -> Multiport Switch1/1
  Multiport Switch1/1 -> Divide1/2
  Sum/1 -> Divide1/1
  Divide1/1 -> Integrator/1
  Constant6/1 -> Multiport Switch1/3
  Constant4/1 -> Multiport Switch1/2
  Constant2/1 -> Multiport Switch/2
  Ttraction/1 -> Multiport Switch/3
  Product2/1 -> Sum/1
  Sign/1 -> Product2/1
  Constant/1 -> Product2/2  "brake torque"
  [V] -> relaxation_length/2(v)  "v"
  relaxation_length/1(slip_relaxed) -> Manual Switch/2
  Divide/1 -> Manual Switch/1, relaxation_length/1(slip_static)  "slip_static"
  Abs/1 -> Divide/2

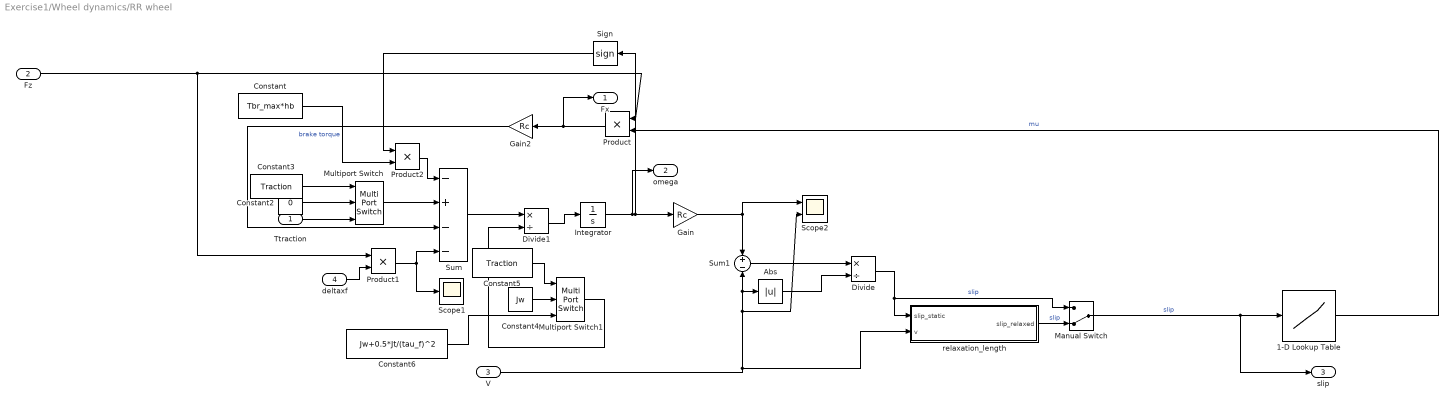
== system Exercise1/Wheel dynamics/RR wheel ==
  Ttraction : Inport
  Fz : Inport  Port=2
  V : Inport  Port=3
  deltaxf : Inport  Port=4
  1-D Lookup Table : Lookup_n-D  NumberOfTableDimensions=1  BreakpointsForDimension1=sigma_vec  Table=mu_vec  InternalRulePriority=Speed  RndMeth=Simplest
  Abs : Abs  SaturateOnIntegerOverflow=off
  Constant : Constant  Value=Tbr_max*hb
  Constant2 : Constant  Value=0
  Constant3 : Constant  Value=Traction
  Constant4 : Constant  Value=Jw
  Constant5 : Constant  Value=Traction
  Constant6 : Constant  Value=Jw+0.5*Jt/(tau_f)^2
  Divide : Product  Inputs=*/
  Divide1 : Product  Inputs=*/
  Gain : Gain  Gain=Rc
  Gain2 : Gain  Gain=Rc
  Integrator : Integrator  InitialCondition=omega0  LimitOutput=on  LowerSaturationLimit=0
  Manual Switch : ManualSwitch  CurrentSetting=0
  Multiport Switch : MultiPortSwitch  Inputs=2  SaturateOnIntegerOverflow=off  InputSameDT=off
  Multiport Switch1 : MultiPortSwitch  Inputs=2  SaturateOnIntegerOverflow=off  InputSameDT=off
  Product : Product
  Product1 : Product
  Product2 : Product
  Scope1 : Scope
      settings: ActiveDisplayYMinimum=1.38626  ActiveDisplayYMaximum=12.08532  DataLoggingVariableName=ScopeData8
  Scope2 : Scope  NumInputPorts=2
      settings: ActiveDisplayYMinimum=-5.62229  ActiveDisplayYMaximum=50.6247  DataLoggingVariableName=ScopeData6
  Sign : Signum
  Sum : Sum  Inputs=-+--
  Sum1 : Sum  Inputs=+-
  relaxation_length : Subsystem
  Fx : Outport
  omega : Outport  Port=2
  slip : Outport  Port=3
  wires:
  Constant/1 -> Product2/2  "brake torque"
  Sign/1 -> Product2/1
  Product2/1 -> Sum/1
  Ttraction/1 -> Multiport Switch/3
  Constant2/1 -> Multiport Switch/2
  Constant4/1 -> Multiport Switch1/2
  Constant6/1 -> Multiport Switch1/3
  Divide1/1 -> Integrator/1
  Sum/1 -> Divide1/1
  Multiport Switch1/1 -> Divide1/2
  Constant5/1 -> Multiport Switch1/1
  Constant3/1 -> Multiport Switch/1
  Multiport Switch/1 -> Sum/2
  Product1/1 -> Scope1/1, Sum/4
  deltaxf/1 -> Product1/2
  Abs/1 -> Divide/2
  Fz/1 -> Product1/1, Product/1
  Manual Switch/1 -> slip/1, 1-D Lookup Table/1  "slip"
  Sum1/1 -> Divide/1
  Integrator/1 -> Sign/1, Gain/1, omega/1
  1-D Lookup Table/1 -> Product/2  "mu"
  Product/1 -> Gain2/1, Fx/1
  V/1 -> relaxation_length/2(v), Scope2/2, Abs/1, Sum1/2
  Gain2/1 -> Sum/3
  Gain/1 -> Scope2/1, Sum1/1
  Divide/1 -> Manual Switch/1, relaxation_length/1(slip_static)  "slip"
  relaxation_length/1(slip_relaxed) -> Manual Switch/2  "slip"

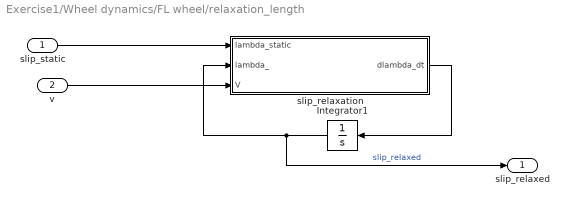
== system Exercise1/Wheel dynamics/FL wheel/relaxation_length ==
  slip_static : Inport
  v : Inport  Port=2
  Integrator1 : Integrator  LimitOutput=on  UpperSaturationLimit=1  LowerSaturationLimit=-1
  slip_relaxation : MATLAB Function  TreatAsAtomicUnit=on
  slip_relaxed : Outport
  wires:
  v/1 -> slip_relaxation/3(V)
  Integrator1/1 -> slip_relaxed/1, slip_relaxation/2(lambda_)  "slip_relaxed"
  slip_relaxation/1(dlambda_dt) -> Integrator1/1
  slip_static/1 -> slip_relaxation/1(lambda_static)

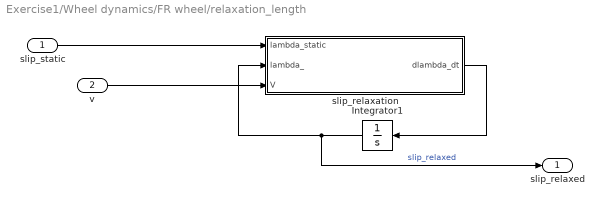
== system Exercise1/Wheel dynamics/FR wheel/relaxation_length ==
  slip_static : Inport
  v : Inport  Port=2
  Integrator1 : Integrator  LimitOutput=on  UpperSaturationLimit=1  LowerSaturationLimit=-1
  slip_relaxation : MATLAB Function  TreatAsAtomicUnit=on
  slip_relaxed : Outport
  wires:
  v/1 -> slip_relaxation/3(V)
  Integrator1/1 -> slip_relaxed/1, slip_relaxation/2(lambda_)  "slip_relaxed"
  slip_relaxation/1(dlambda_dt) -> Integrator1/1
  slip_static/1 -> slip_relaxation/1(lambda_static)

== system Exercise1/Wheel dynamics/RL wheel/relaxation_length ==
  slip_static : Inport
  v : Inport  Port=2
  Integrator1 : Integrator  LimitOutput=on  UpperSaturationLimit=1  LowerSaturationLimit=-1
  slip_relaxation : MATLAB Function  TreatAsAtomicUnit=on
  slip_relaxed : Outport
  wires:
  v/1 -> slip_relaxation/3(V)
  Integrator1/1 -> slip_relaxed/1, slip_relaxation/2(lambda_)  "slip_relaxed"
  slip_relaxation/1(dlambda_dt) -> Integrator1/1
  slip_static/1 -> slip_relaxation/1(lambda_static)

== system Exercise1/Wheel dynamics/RR wheel/relaxation_length ==
  slip_static : Inport
  v : Inport  Port=2
  Integrator1 : Integrator  LimitOutput=on  UpperSaturationLimit=1  LowerSaturationLimit=-1
  slip_relaxation : MATLAB Function  TreatAsAtomicUnit=on
  slip_relaxed : Outport
  wires:
  v/1 -> slip_relaxation/3(V)
  Integrator1/1 -> slip_relaxed/1, slip_relaxation/2(lambda_)  "slip_relaxed"
  slip_relaxation/1(dlambda_dt) -> Integrator1/1
  slip_static/1 -> slip_relaxation/1(lambda_static)

== matlab function Exercise1/Wheel dynamics/FL wheel/relaxation_length/slip_relaxation ==
  data: lambda_static input; dlambda_dt output; lambda_ input; V input
function dlambda_dt = fcn(lambda_static, lambda_, V )

sigma = 0.05;   % Relaxation length (m) 

if V > 1
    dlambda_dt = (V / sigma) * (lambda_static - lambda_);
else 
    dlambda_dt = -lambda_/0.1;  % Decay to zero if stopped
end

== matlab function Exercise1/Gear shifting logic/Gear shifting logic ==
  data: omega_t input; gearRatio output; gN_vect input; shiftspeed input; gear output; gearPrevious input
function [gearRatio, gear] = fcn(omega_t, gN_vect, shiftspeed, gearPrevious)
gearRatio = gN_vect(gearPrevious);
gear = gearPrevious;
    if ( omega_t*gearRatio > shiftspeed(1)) && gearPrevious < length(gN_vect)
    %if ( omega_w*gearRatio > shiftspeed(1)) && gearPrevious < length(gN_vect) %omega_t*gearRatio > shiftspeed(1) ||
        gear = gearPrevious+1;
        gearRatio = gN_vect(gear);
    elseif omega_t*gearRatio < shiftspeed(2) && gearPrevious > 1
        gear = gearPrevious-1;
        gearRatio = gN_vect(gear);
    end
end

== matlab function Exercise1/Gear shifting logic/MATLAB Function ==
  data: hc output; trigger input; t input; t_step input; tNext output; t_pedalAct input; t_shifting input
function [hc, tNext] = fcn(trigger,t, t_step,t_pedalAct, t_shifting)
tNext = t+t_step;
    if trigger
        tNext = 0;
        hc = 1;
    else
        hc = 1+1./(1+exp(15*(t-t_pedalAct/2)))-1./(1+exp(15*(t-t_shifting-3*t_pedalAct/2)));
    end
end

% hc represents a smooth modulation factor on the clutch command during a gear shift. 
% It reduces clutch command during the shift, then restores it afterward.

== matlab function Exercise1/Engine + clutch1/Clutch1 ==
  data: u input; Tc output; Tcmax input; Temax input; hc input; ha input
function Tc = fcn(u, Tcmax, Temax, hc, ha)
Tc = ha*Temax;
if Temax < 0
    Tc = Temax;
end
if u > 0
    Tc = hc*Tcmax;
elseif u < 0
    Tc = -hc*Tcmax;
end
end

== matlab function Exercise1/Wheel dynamics/RL wheel/relaxation_length/slip_relaxation ==
  data: lambda_static input; dlambda_dt output; lambda_ input; V input
function dlambda_dt = fcn(lambda_static, lambda_, V )

sigma = 0.05;   % Relaxation length (m) 

if V > 0.1
    dlambda_dt = (V / sigma) * (lambda_static - lambda_);
else 
    dlambda_dt = -lambda_/0.1;  % Decay to zero if stopped
end

== matlab function Exercise1/Wheel dynamics/FR wheel/relaxation_length/slip_relaxation ==
  data: lambda_static input; dlambda_dt output; lambda_ input; V input
function dlambda_dt = fcn(lambda_static, lambda_, V )

sigma = 0.05;   % Relaxation length (m) 

if V > 0.1
    dlambda_dt = (V / sigma) * (lambda_static - lambda_);
else 
    dlambda_dt = -lambda_/0.1;  % Decay to zero if stopped
end

== matlab function Exercise1/Wheel dynamics/RR wheel/relaxation_length/slip_relaxation ==
  data: lambda_static input; dlambda_dt output; lambda_ input; V input
function dlambda_dt = fcn(lambda_static, lambda_, V )

sigma = 0.05;   % Relaxation length (m) 

if V > 0.1
    dlambda_dt = (V / sigma) * (lambda_static - lambda_);
else 
    dlambda_dt = -lambda_/0.1;  % Decay to zero if stopped
end
